simulink model "SIRVHDB_MPC_model"  (R2025a)
settings: Solver=VariableStepAuto  StartTime=0.0  StopTime=1500  RelTol=1e-3
values from neighbouring files (symbols this model uses):
  beta1 = 0.45    [SIRVDB_model_parameters.m]
  beta2 = 0.45    [SIRVDB_model_parameters.m]
  epsilon = 0.6    [SIRVDB_model_parameters.m]
  eta = 0.6    [SIRVDB_model_parameters.m]
  gamma = 1/12    (= 0.0833333333333)    [SIRVDB_model_parameters.m]
  gamma_h = 1/25    (= 0.04)    [SIRVDB_model_parameters.m]
  gamma_v = 1/9    (= 0.111111111111)    [SIRVDB_model_parameters.m]
  h = 0.05    [SIRVDB_model_parameters.m]
  H_cap1 = 0.005    [SIRVDB_model_parameters.m]
  H_cap2 = 0.005    [SIRVDB_model_parameters.m]
  H_ref = 0.8 * (H_cap1 + H_cap2)    (= 0.008)    [SIRVDB_model_parameters.m]
  h_v = 0.02    [SIRVDB_model_parameters.m]
  k = 0.7    [SIRVDB_model_parameters.m]
  M11 = 0.85    [SIRVDB_model_parameters.m]
  M12 = 0.15    [SIRVDB_model_parameters.m]
  M21 = 0.10    (= 0.1)    [SIRVDB_model_parameters.m]
  M22 = 0.90    (= 0.9)    [SIRVDB_model_parameters.m]
  mu = 0.001    [SIRVDB_model_parameters.m]
  mu_h = 0.02    [SIRVDB_model_parameters.m]
  mu_v = 0.0005    [SIRVDB_model_parameters.m]
  nu1 = 0    [SIRVDB_model_parameters.m]
  nu2 = 0    [SIRVDB_model_parameters.m]
  omega_R = 1/110    (= 0.00909090909091)    [SIRVDB_model_parameters.m]
  omega_V = 1/140    (= 0.00714285714286)    [SIRVDB_model_parameters.m]
  season_amp = 0.4    [SIRVDB_model_parameters.m]
  season_period = 365    [SIRVDB_model_parameters.m]
  travel = [-0.02  0.02 ... (first row only)    [SIRVDB_model_parameters.m]
  u1 = 0    [SIRVDB_model_parameters.m]
  u2 = 0    [SIRVDB_model_parameters.m]
libraries: mpclib x1
settings Model: Creator=Hakon  LastModifiedBy=welde
settings RTWCC: GPUComputeCapability=3.5

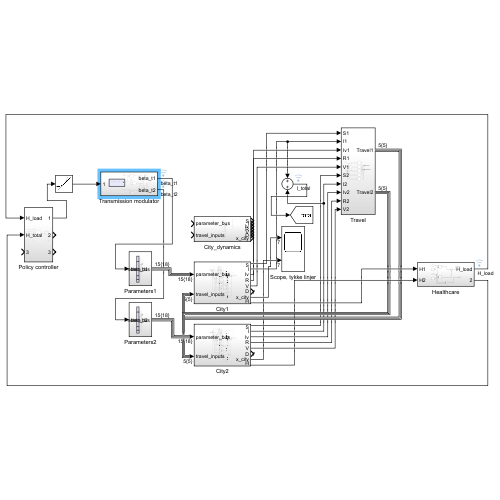
[thumbnail: Simulink's stored preview of the top-level diagram]
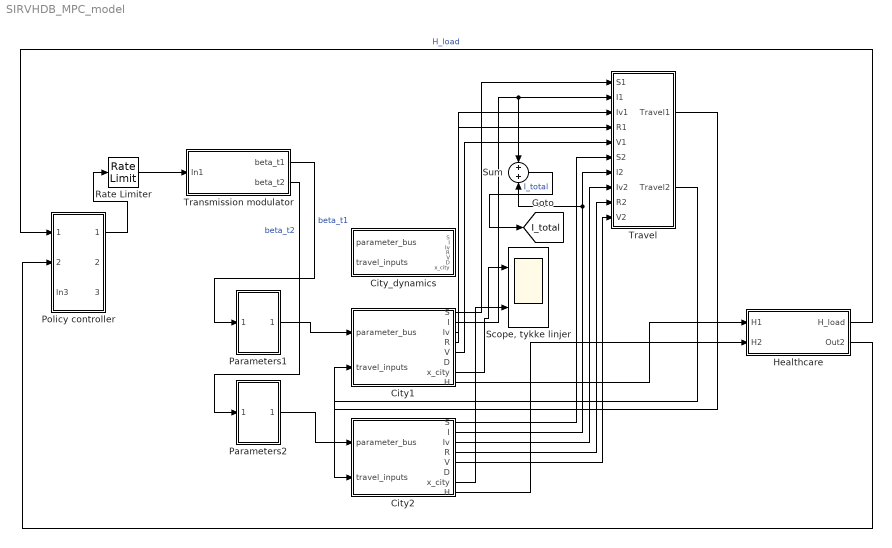
== system SIRVHDB_MPC_model ==
  City1 : Subsystem
  City2 : Subsystem
  City_dynamics : Subsystem
  Healthcare : Subsystem
  Parameters1 : Subsystem
  Parameters2 : Subsystem
  Policy controller : Subsystem
  Rate Limiter : RateLimiter  RisingSlewLimit=0.05  FallingSlewLimit=-0.05  SampleTimeMode=inherited
  "Scope, tykke linjer" : Scope  NumInputPorts=2
      settings: ActiveDisplayYMinimum=-0.125  ActiveDisplayYMaximum=1.125
  Sum : Sum
  Transmission modulator : Subsystem
  Travel : Subsystem
  tag scope: I_total=global
  wires:
  Parameters1/1(parameter_bus) -> City1/1(parameter_bus)
  City1/7(x_city) -> "Scope, tykke linjer"/1
  City2/7(x_city) -> "Scope, tykke linjer"/2
  Parameters2/1(parameter_bus) -> City2/1(parameter_bus)
  City1/1(S) -> Travel/1(S1)
  City1/2(I) -> Travel/2(I1), Sum/1
  City1/3(Iv) -> Travel/3(Iv1)
  City1/4(R) -> Travel/4(R1)
  City1/5(V) -> Travel/5(V1)
  City2/1(S) -> Travel/6(S2)
  City2/2(I) -> Travel/7(I2), Sum/2
  City2/3(Iv) -> Travel/8(Iv2)
  City2/4(R) -> Travel/9(R2)
  City2/5(V) -> Travel/10(V2)
  Travel/1(Travel1) -> City1/2(travel_inputs)
  Travel/2(Travel2) -> City2/2(travel_inputs)
  City1/8(H) -> Healthcare/1(H1)
  City2/8(H) -> Healthcare/2(H2)
  Healthcare/1(H_load) -> Policy controller/1(H_load)  "H_load"
  Transmission modulator/1(beta_t1) -> Parameters1/1(beta_t1)  "beta_t1"
  Transmission modulator/2(beta_t2) -> Parameters2/1(beta_t2)  "beta_t2"
  Healthcare/2(Out2) -> Policy controller/2(H_total)
  Policy controller/1(Out1) -> Rate Limiter/1
  Rate Limiter/1 -> Transmission modulator/1(In1)
  Sum/1 -> [I_total]  "I_total"

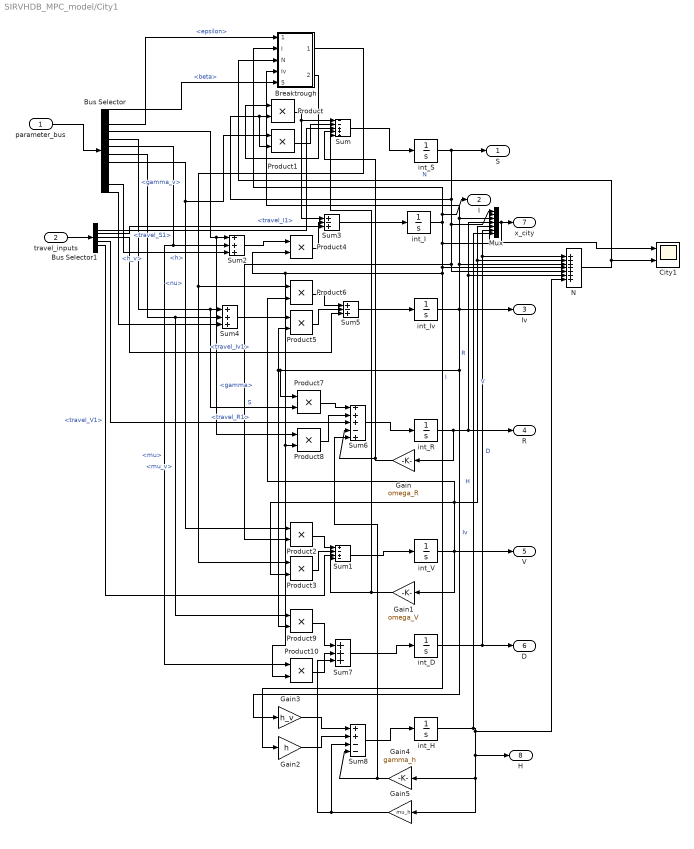
== system SIRVHDB_MPC_model/City1 ==
  parameter_bus : Inport
  travel_inputs : Inport  Port=2
  Breaktrough : Subsystem
  Bus Selector : BusSelector  OutputSignals=beta,eta,epsilon,gamma,gamma_v,mu,mu_v,nu,omega_V,omega_R,h,h_v
  Bus Selector1 : BusSelector  OutputSignals=travel_S1,travel_I1,travel_Iv1,travel_R1,travel_V1
  City1 : Scope  NumInputPorts=2
      settings: ActiveDisplayYMinimum=-0.12499999999999997  ActiveDisplayYMaximum=1.125
  Gain : Gain  Gain=omega_R
  Gain1 : Gain  Gain=omega_V
  Gain2 : Gain  Gain=h
  Gain3 : Gain  Gain=h_v
  Gain4 : Gain  Gain=gamma_h
  Gain5 : Gain  Gain=mu_h
  Mux : Mux  Inputs=7
  N : Sum  Inputs=+++++++
  Product{,1..10} (11 alike) : Product
  Sum : Sum  Inputs=--+++
  Sum1 : Sum  Inputs=+-+-
  Sum2 : Sum  Inputs=+++
  Sum3 : Sum  Inputs=+-+
  Sum4 : Sum  Inputs=+++
  Sum5 : Sum  Inputs=+-+
  Sum6 : Sum  Inputs=+++-+
  Sum7 : Sum  Inputs=+++
  Sum8 : Sum  Inputs=++--
  int_D : Integrator
  int_H : Integrator
  int_I : Integrator  InitialCondition=0.01
  int_Iv : Integrator
  int_R : Integrator
  int_S : Integrator  InitialCondition=0.99
  int_V : Integrator
  S : Outport
  I : Outport  Port=2
  Iv : Outport  Port=3
  R : Outport  Port=4
  V : Outport  Port=5
  D : Outport  Port=6
  x_city : Outport  Port=7
  H : Outport  Port=8
  wires:
  int_S/1 -> S/1, Product2/2, N/5, Mux/1, Product1/2, Product/2  "S"
  int_I/1 -> Gain2/1, Product8/2, Product10/2, Product4/2, N/4, Mux/2, I/1, Breaktrough/2(I)  "I"
  int_Iv/1 -> Gain3/1, Product9/2, Product5/2, Product7/1, Iv/1, Breaktrough/4(Iv), Mux/3, N/3  "Iv"
  int_R/1 -> Gain/1, R/1, N/6, Mux/4  "R"
  int_V/1 -> Gain1/1, V/1, Product6/2, Product3/2, Mux/5, N/2  "V"
  int_D/1 -> D/1, Mux/6, N/1  "D"
  Mux/1 -> City1/1, x_city/1
  parameter_bus/1 -> Bus Selector/1
  Bus Selector/3 -> Breaktrough/1(<epsilon>)  "<epsilon>"
  N/1 -> City1/2, Breaktrough/3(N)  "N"
  Breaktrough/2(lambda) -> Product/1
  Bus Selector/8 -> Product2/1, Product1/1  "<nu>"
  Product/1 -> Sum3/1, Sum/1
  Product1/1 -> Sum/2
  Sum/1 -> int_S/1
  Breaktrough/1(lambda_v) -> Product6/1, Product3/1
  Product2/1 -> Sum1/1
  Product3/1 -> Sum1/2
  Sum1/1 -> int_V/1
  Bus Selector/7 -> Product9/1, Sum4/2  "<mu_v>"
  Bus Selector/4 -> Product8/1, Sum2/1  "<gamma>"
  Sum2/1 -> Product4/1
  Product4/1 -> Sum3/2
  Sum3/1 -> int_I/1
  Bus Selector/5 -> Product7/2, Sum4/1  "<gamma_v>"
  Bus Selector/6 -> Product10/1, Sum2/2  "<mu>"
  Product5/1 -> Sum5/2
  Sum4/1 -> Product5/1
  Product6/1 -> Sum5/1
  Sum5/1 -> int_Iv/1
  Sum6/1 -> int_R/1
  Product7/1 -> Sum6/1
  Product8/1 -> Sum6/2
  Product9/1 -> Sum7/1
  Product10/1 -> Sum7/2
  Sum7/1 -> int_D/1
  travel_inputs/1 -> Bus Selector1/1
  Bus Selector1/1 -> Sum/3  "<travel_S1>"
  Bus Selector1/2 -> Sum3/3  "<travel_I1>"
  Bus Selector1/3 -> Sum5/3  "<travel_Iv1>"
  Bus Selector1/4 -> Sum6/3  "<travel_R1>"
  Bus Selector1/5 -> Sum1/3  "<travel_V1>"
  Gain/1 -> Sum/4, Sum6/4
  Gain1/1 -> Sum1/4, Sum/5
  int_H/1 -> Mux/7, N/7, H/1, Gain5/1, Gain4/1  "H"
  Sum8/1 -> int_H/1
  Gain2/1 -> Sum8/2
  Gain3/1 -> Sum8/1
  Gain4/1 -> Sum6/5, Sum8/4
  Gain5/1 -> Sum7/3, Sum8/3
  Bus Selector/11 -> Sum2/3  "<h>"
  Bus Selector/12 -> Sum4/3  "<h_v>"
  Bus Selector/1 -> Breaktrough/5(<beta>)  "<beta>"

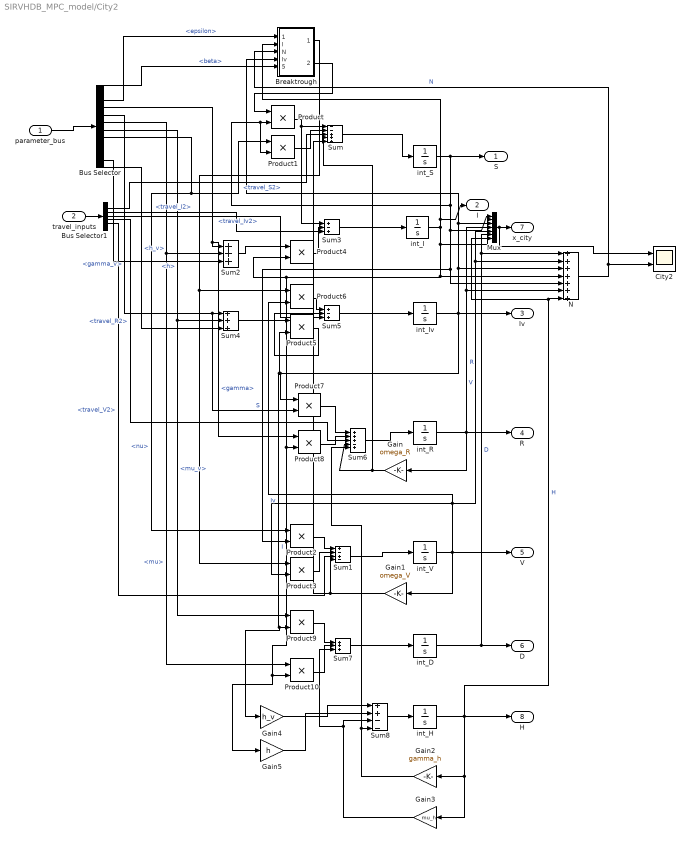
== system SIRVHDB_MPC_model/City2 ==
  parameter_bus : Inport
  travel_inputs : Inport  Port=2
  Breaktrough : Subsystem
  Bus Selector : BusSelector  OutputSignals=beta,eta,epsilon,gamma,gamma_v,mu,mu_v,nu,omega_V,omega_R,h,h_v
  Bus Selector1 : BusSelector  OutputSignals=travel_S2,travel_I2,travel_Iv2,travel_R2,travel_V2
  City2 : Scope  NumInputPorts=2
      settings: ActiveDisplayYMinimum=-0.125  ActiveDisplayYMaximum=1.125
  Gain : Gain  Gain=omega_R
  Gain1 : Gain  Gain=omega_V
  Gain2 : Gain  Gain=gamma_h
  Gain3 : Gain  Gain=mu_h
  Gain4 : Gain  Gain=h_v
  Gain5 : Gain  Gain=h
  Mux : Mux  Inputs=7
  N : Sum  Inputs=+++++++
  Product{,1..10} (11 alike) : Product
  Sum : Sum  Inputs=--+++
  Sum1 : Sum  Inputs=+-+-
  Sum2 : Sum  Inputs=+++
  Sum3 : Sum  Inputs=+-+
  Sum4 : Sum  Inputs=+++
  Sum5 : Sum  Inputs=+-+
  Sum6 : Sum  Inputs=+++-+
  Sum7 : Sum  Inputs=+++
  Sum8 : Sum  Inputs=++--
  int_D : Integrator
  int_H : Integrator
  int_I : Integrator  InitialCondition=0.01
  int_Iv : Integrator
  int_R : Integrator
  int_S : Integrator  InitialCondition=0.99
  int_V : Integrator
  S : Outport
  I : Outport  Port=2
  Iv : Outport  Port=3
  R : Outport  Port=4
  V : Outport  Port=5
  D : Outport  Port=6
  x_city : Outport  Port=7
  H : Outport  Port=8
  wires:
  int_S/1 -> S/1, Product2/2, N/5, Mux/1, Product1/2, Product/2  "S"
  int_I/1 -> Product8/2, Gain5/1, Product10/2, Product4/2, N/4, Mux/2, I/1, Breaktrough/2(I)  "I"
  int_Iv/1 -> Iv/1, Gain4/1, Product9/2, Product5/2, Product7/1, Breaktrough/4(Iv), Mux/3, N/3  "Iv"
  int_R/1 -> Gain/1, R/1, Mux/4, N/6  "R"
  int_V/1 -> Gain1/1, V/1, Product6/2, Product3/2, Mux/5, N/2  "V"
  int_D/1 -> D/1, Mux/6, N/1  "D"
  Mux/1 -> City2/1, x_city/1
  parameter_bus/1 -> Bus Selector/1
  Bus Selector/3 -> Breaktrough/1(<epsilon>)  "<epsilon>"
  N/1 -> City2/2, Breaktrough/3(N)  "N"
  Breaktrough/2(lambda) -> Product/1
  Bus Selector/8 -> Product2/1, Product1/1  "<nu>"
  Product/1 -> Sum3/1, Sum/1
  Product1/1 -> Sum/2
  Breaktrough/1(lambda_v) -> Product6/1, Product3/1
  Product2/1 -> Sum1/1
  Product3/1 -> Sum1/2
  Sum1/1 -> int_V/1
  Bus Selector/7 -> Product9/1, Sum4/2  "<mu_v>"
  Bus Selector/4 -> Product8/1, Sum2/1  "<gamma>"
  Sum2/1 -> Product4/1
  Product4/1 -> Sum3/2
  Sum3/1 -> int_I/1
  Bus Selector/5 -> Product7/2, Sum4/1  "<gamma_v>"
  Bus Selector/6 -> Product10/1, Sum2/2  "<mu>"
  Product5/1 -> Sum5/2
  Sum4/1 -> Product5/1
  Product6/1 -> Sum5/1
  Sum5/1 -> int_Iv/1
  Sum6/1 -> int_R/1
  Product7/1 -> Sum6/1
  Product8/1 -> Sum6/2
  Product9/1 -> Sum7/1
  Product10/1 -> Sum7/2
  Sum7/1 -> int_D/1
  travel_inputs/1 -> Bus Selector1/1
  Bus Selector1/1 -> Sum/3  "<travel_S2>"
  Bus Selector1/2 -> Sum3/3  "<travel_I2>"
  Bus Selector1/3 -> Sum5/3  "<travel_Iv2>"
  Bus Selector1/4 -> Sum6/3  "<travel_R2>"
  Bus Selector1/5 -> Sum1/3  "<travel_V2>"
  Gain/1 -> Sum6/4, Sum/4
  Gain1/1 -> Sum/5, Sum1/4
  Bus Selector/11 -> Sum2/3  "<h>"
  Bus Selector/12 -> Sum4/3  "<h_v>"
  int_H/1 -> Mux/7, N/7, H/1, Gain3/1, Gain2/1  "H"
  Sum8/1 -> int_H/1
  Gain2/1 -> Sum6/5, Sum8/4
  Gain3/1 -> Sum7/3, Sum8/3
  Gain4/1 -> Sum8/1
  Gain5/1 -> Sum8/2
  Bus Selector/1 -> Breaktrough/5(beta_t2)  "<beta>"
  Sum/1 -> int_S/1

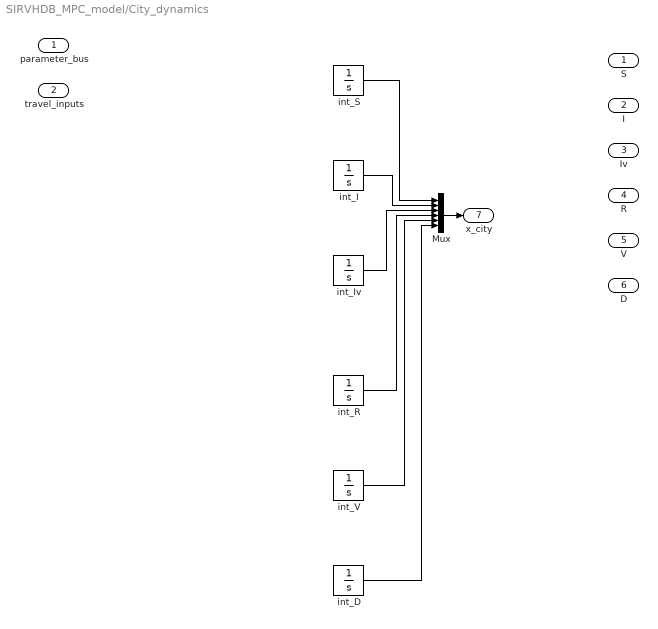
== system SIRVHDB_MPC_model/City_dynamics ==
  parameter_bus : Inport
  travel_inputs : Inport  Port=2
  Mux : Mux  Inputs=6
  int_D : Integrator
  int_I : Integrator  InitialCondition=0.01
  int_Iv : Integrator
  int_R : Integrator
  int_S : Integrator  InitialCondition=0.99
  int_V : Integrator
  S : Outport
  I : Outport  Port=2
  Iv : Outport  Port=3
  R : Outport  Port=4
  V : Outport  Port=5
  D : Outport  Port=6
  x_city : Outport  Port=7
  wires:
  int_S/1 -> Mux/1
  int_I/1 -> Mux/2
  int_Iv/1 -> Mux/3
  int_R/1 -> Mux/4
  int_V/1 -> Mux/5
  int_D/1 -> Mux/6
  Mux/1 -> x_city/1

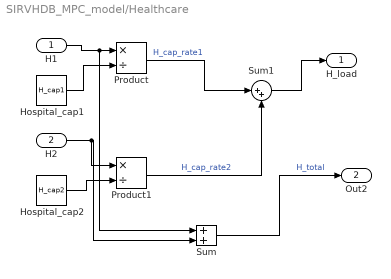
== system SIRVHDB_MPC_model/Healthcare ==
  H1 : Inport
  H2 : Inport  Port=2
  Hospital_cap1 : Constant  Value=H_cap1
  Hospital_cap2 : Constant  Value=H_cap2
  Product : Product  Inputs=*/
  Product1 : Product  Inputs=*/
  Sum : Sum
  Sum1 : Sum  Inputs=|++
  H_load : Outport
  Out2 : Outport  Port=2
  wires:
  H2/1 -> Sum/2, Product1/1
  Hospital_cap2/1 -> Product1/2
  H1/1 -> Sum/1, Product/1
  Hospital_cap1/1 -> Product/2
  Product/1 -> Sum1/1  "H_cap_rate1"
  Product1/1 -> Sum1/2  "H_cap_rate2"
  Sum1/1 -> H_load/1
  Sum/1 -> Out2/1  "H_total"

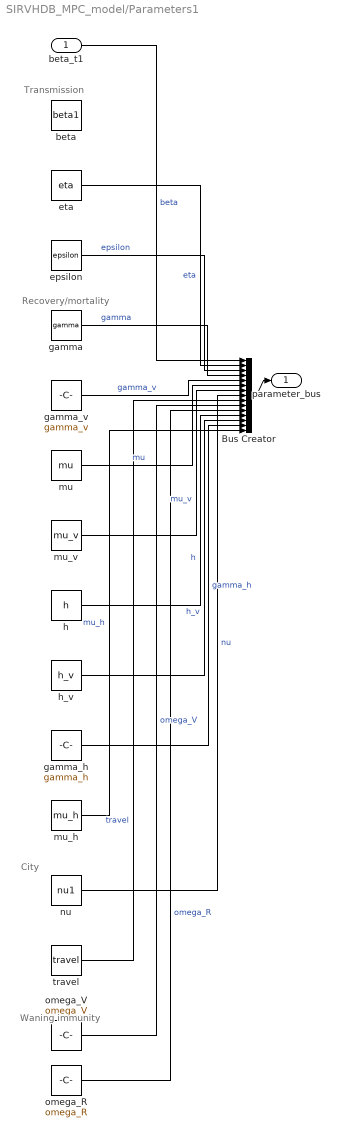
== system SIRVHDB_MPC_model/Parameters1 ==
  note: Waning immunity
  note: Transmission
  note: City
  note: Recovery/mortality
  beta_t1 : Inport
  Bus Creator : BusCreator  Inputs=15
  beta : Constant  Value=beta1  SampleTime=-1
  epsilon : Constant  Value=epsilon  SampleTime=-1
  eta : Constant  Value=eta  SampleTime=-1
  gamma : Constant  Value=gamma  SampleTime=-1
  gamma_h : Constant  Value=gamma_h  SampleTime=-1
  gamma_v : Constant  Value=gamma_v  SampleTime=-1
  h : Constant  Value=h  SampleTime=-1
  h_v : Constant  Value=h_v  SampleTime=-1
  mu : Constant  Value=mu  SampleTime=-1
  mu_h : Constant  Value=mu_h  SampleTime=-1
  mu_v : Constant  Value=mu_v  SampleTime=-1
  nu : Constant  Value=nu1  SampleTime=-1
  omega_R : Constant  Value=omega_R  SampleTime=-1
  omega_V : Constant  Value=omega_V  SampleTime=-1
  travel : Constant  Value=travel  SampleTime=-1
  parameter_bus : Outport
  wires:
  travel/1 -> Bus Creator/9  "travel"
  mu_v/1 -> Bus Creator/7  "mu_v"
  Bus Creator/1 -> parameter_bus/1
  epsilon/1 -> Bus Creator/3  "epsilon"
  eta/1 -> Bus Creator/2  "eta"
  gamma/1 -> Bus Creator/4  "gamma"
  nu/1 -> Bus Creator/8  "nu"
  gamma_v/1 -> Bus Creator/5  "gamma_v"
  mu/1 -> Bus Creator/6  "mu"
  omega_V/1 -> Bus Creator/10  "omega_V"
  omega_R/1 -> Bus Creator/11  "omega_R"
  beta_t1/1 -> Bus Creator/1  "beta"
  h/1 -> Bus Creator/12  "h"
  h_v/1 -> Bus Creator/13  "h_v"
  gamma_h/1 -> Bus Creator/14  "gamma_h"
  mu_h/1 -> Bus Creator/15  "mu_h"

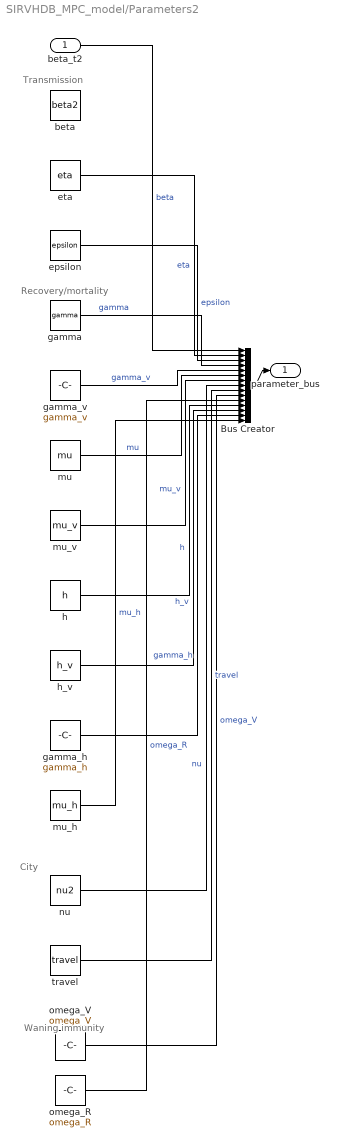
== system SIRVHDB_MPC_model/Parameters2 ==
  note: Transmission
  note: City
  note: Recovery/mortality
  note: Waning immunity
  beta_t2 : Inport
  Bus Creator : BusCreator  Inputs=15
  beta : Constant  Value=beta2  SampleTime=-1
  epsilon : Constant  Value=epsilon  SampleTime=-1
  eta : Constant  Value=eta  SampleTime=-1
  gamma : Constant  Value=gamma  SampleTime=-1
  gamma_h : Constant  Value=gamma_h  SampleTime=-1
  gamma_v : Constant  Value=gamma_v  SampleTime=-1
  h : Constant  Value=h  SampleTime=-1
  h_v : Constant  Value=h_v  SampleTime=-1
  mu : Constant  Value=mu  SampleTime=-1
  mu_h : Constant  Value=mu_h  SampleTime=-1
  mu_v : Constant  Value=mu_v  SampleTime=-1
  nu : Constant  Value=nu2  SampleTime=-1
  omega_R : Constant  Value=omega_R  SampleTime=-1
  omega_V : Constant  Value=omega_V  SampleTime=-1
  travel : Constant  Value=travel  SampleTime=-1
  parameter_bus : Outport
  wires:
  travel/1 -> Bus Creator/9  "travel"
  mu_v/1 -> Bus Creator/7  "mu_v"
  Bus Creator/1 -> parameter_bus/1
  epsilon/1 -> Bus Creator/3  "epsilon"
  eta/1 -> Bus Creator/2  "eta"
  gamma/1 -> Bus Creator/4  "gamma"
  nu/1 -> Bus Creator/8  "nu"
  gamma_v/1 -> Bus Creator/5  "gamma_v"
  mu/1 -> Bus Creator/6  "mu"
  omega_V/1 -> Bus Creator/10  "omega_V"
  omega_R/1 -> Bus Creator/11  "omega_R"
  beta_t2/1 -> Bus Creator/1  "beta"
  h/1 -> Bus Creator/12  "h"
  h_v/1 -> Bus Creator/13  "h_v"
  gamma_h/1 -> Bus Creator/14  "gamma_h"
  mu_h/1 -> Bus Creator/15  "mu_h"

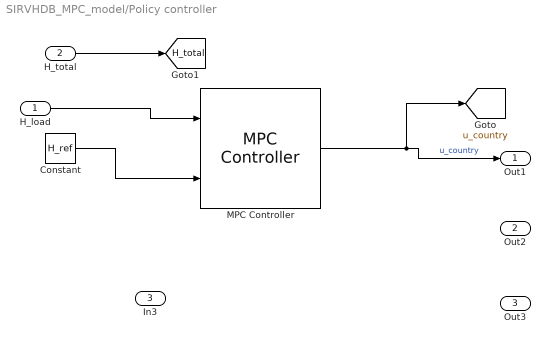
== system SIRVHDB_MPC_model/Policy controller ==
  H_load : Inport
  H_total : Inport  Port=2
  In3 : Inport  Port=3
  Constant : Constant  Value=H_ref  SampleTime=-1
  MPC Controller : mpclib/MPC Controller  SCDEnableBlockLinearizationSpecification=on  mpcobj=mpcobj  x0=xmpc  is_multiple=0  enable_value=0  return_u0=off  updateMPCinCallerWorkspace=on  md_inport=off  mv_inport=off  uref_inport=off  return_cost=off  return_mvseq=off  return_qpstatus=off  return_xseq=off  return_state=off  return_ovseq=off  state_inport=off  umin_inport=off  umax_inport=off  ymin_inport=off  ymax_inport=off  cc_inport=off  ywt_inport=off  uwt_inport=off  duwt_inport=off  rhoeps_inport=off  pm_inport=off  MaximumP=10  HorizonChoice=FixedHorizon  n_ts=1  n_p=40  n_mv=1  n_md=0  n_ud=0  n_mo=1  n_uo=0  BlockDataType=double  SampleTimeInherited=off  switch_inport=off
  Out1 : Outport
  Out2 : Outport  Port=2
  Out3 : Outport  Port=3
  tag scope: H_total=global, u_country=global
  wires:
  ? -> Out2/1
  ? -> Out3/1
  H_total/1 -> [H_total]
  H_load/1 -> MPC Controller/1
  MPC Controller/1 -> [u_country], Out1/1  "u_country"
  Constant/1 -> MPC Controller/2

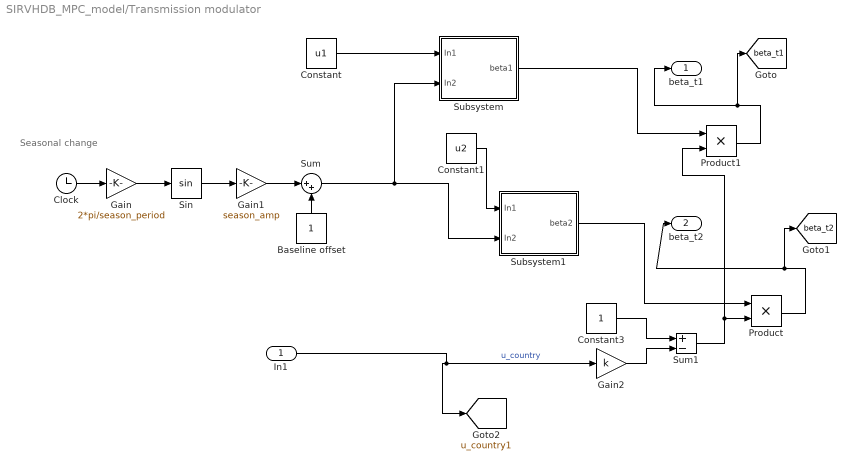
== system SIRVHDB_MPC_model/Transmission modulator ==
  note: Seasonal change
  In1 : Inport
  Baseline offset : Constant  SampleTime=-1
  Clock : Clock
  Constant : Constant  Value=u1
  Constant1 : Constant  Value=u2
  Constant3 : Constant
  Gain : Gain  Gain=2*pi/season_period
  Gain1 : Gain  Gain=season_amp
  Gain2 : Gain  Gain=k
  Product : Product
  Product1 : Product
  Sin : Trigonometry
  Subsystem : Subsystem
  Subsystem1 : Subsystem
  Sum : Sum  Inputs=|++
  Sum1 : Sum  Inputs=+-
  beta_t1 : Outport
  beta_t2 : Outport  Port=2
  tag scope: beta_t1=global, beta_t2=global, u_country1=global
  wires:
  Gain1/1 -> Sum/1
  Baseline offset/1 -> Sum/2
  Gain/1 -> Sin/1
  Sin/1 -> Gain1/1
  Clock/1 -> Gain/1
  Constant/1 -> Subsystem/1(In1)
  Sum/1 -> Subsystem1/2(In2), Subsystem/2(In2)
  Subsystem/1(beta1) -> Product1/1
  Constant1/1 -> Subsystem1/1(In1)
  Subsystem1/1(beta2) -> Product/1
  In1/1 -> Gain2/1, [u_country1]  "u_country"
  Gain2/1 -> Sum1/2
  Constant3/1 -> Sum1/1
  Sum1/1 -> Product1/2, Product/2
  Product/1 -> [beta_t2], beta_t2/1
  Product1/1 -> [beta_t1], beta_t1/1

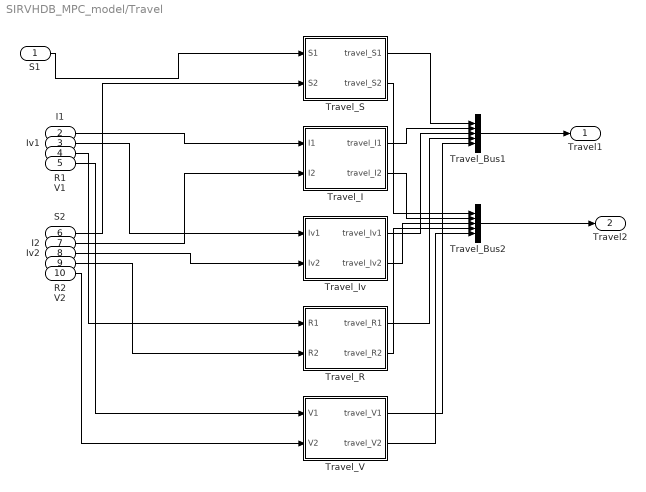
== system SIRVHDB_MPC_model/Travel ==
  S1 : Inport
  I1 : Inport  Port=2
  Iv1 : Inport  Port=3
  R1 : Inport  Port=4
  V1 : Inport  Port=5
  S2 : Inport  Port=6
  I2 : Inport  Port=7
  Iv2 : Inport  Port=8
  R2 : Inport  Port=9
  V2 : Inport  Port=10
  Travel_Bus1 : BusCreator  Inputs=5
  Travel_Bus2 : BusCreator  Inputs=5
  Travel_I : Subsystem
  Travel_Iv : Subsystem
  Travel_R : Subsystem
  Travel_S : Subsystem
  Travel_V : Subsystem
  Travel1 : Outport
  Travel2 : Outport  Port=2
  wires:
  Travel_Bus2/1 -> Travel2/1
  V1/1 -> Travel_V/1(V1)
  S2/1 -> Travel_S/2(S2)
  V2/1 -> Travel_V/2(V2)
  Iv1/1 -> Travel_Iv/1(Iv1)
  Travel_V/2(travel_V2) -> Travel_Bus2/5
  Travel_Iv/2(travel_Iv2) -> Travel_Bus2/3
  Travel_I/2(travel_I2) -> Travel_Bus2/2
  Travel_R/2(travel_R2) -> Travel_Bus2/4
  I1/1 -> Travel_I/1(I1)
  Travel_I/1(travel_I1) -> Travel_Bus1/2
  I2/1 -> Travel_I/2(I2)
  Iv2/1 -> Travel_Iv/2(Iv2)
  Travel_Bus1/1 -> Travel1/1
  Travel_S/1(travel_S1) -> Travel_Bus1/1
  R1/1 -> Travel_R/1(R1)
  Travel_Iv/1(travel_Iv1) -> Travel_Bus1/3
  R2/1 -> Travel_R/2(R2)
  Travel_S/2(travel_S2) -> Travel_Bus2/1
  Travel_R/1(travel_R1) -> Travel_Bus1/4
  Travel_V/1(travel_V1) -> Travel_Bus1/5
  S1/1 -> Travel_S/1(S1)

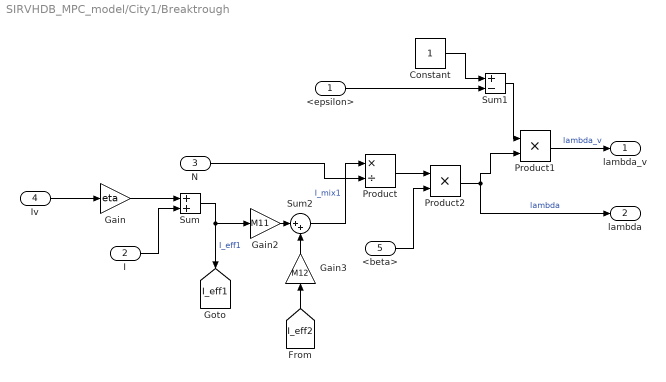
== system SIRVHDB_MPC_model/City1/Breaktrough ==
  <epsilon> : Inport
  I : Inport  Port=2
  N : Inport  Port=3
  Iv : Inport  Port=4
  <beta> : Inport  Port=5
  Constant : Constant
  Gain : Gain  Gain=eta
  Gain2 : Gain  Gain=M11
  Gain3 : Gain  Gain=M12
  Product : Product  Inputs=*/
  Product1 : Product
  Product2 : Product
  Sum : Sum
  Sum1 : Sum  Inputs=+-
  Sum2 : Sum  Inputs=|++
  lambda_v : Outport
  lambda : Outport  Port=2
  tag scope: I_eff1=global
  wires:
  Product1/1 -> lambda_v/1  "lambda_v"
  <epsilon>/1 -> Sum1/2
  Gain/1 -> Sum/1
  I/1 -> Sum/2
  Product2/1 -> Product1/2, lambda/1  "lambda"
  Constant/1 -> Sum1/1
  Product/1 -> Product2/1
  N/1 -> Product/2
  Sum/1 -> [I_eff1], Gain2/1  "I_eff1"
  Iv/1 -> Gain/1
  Sum1/1 -> Product1/1
  [I_eff2] -> Gain3/1
  Gain2/1 -> Sum2/1
  Gain3/1 -> Sum2/2
  Sum2/1 -> Product/1  "I_mix1"
  <beta>/1 -> Product2/2

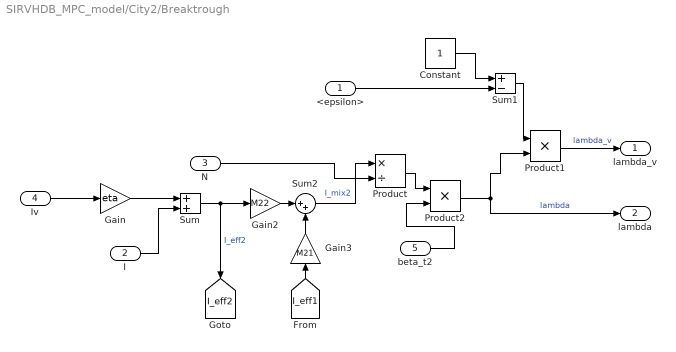
== system SIRVHDB_MPC_model/City2/Breaktrough ==
  <epsilon> : Inport
  I : Inport  Port=2
  N : Inport  Port=3
  Iv : Inport  Port=4
  beta_t2 : Inport  Port=5
  Constant : Constant
  Gain : Gain  Gain=eta
  Gain2 : Gain  Gain=M22
  Gain3 : Gain  Gain=M21
  Product : Product  Inputs=*/
  Product1 : Product
  Product2 : Product
  Sum : Sum
  Sum1 : Sum  Inputs=+-
  Sum2 : Sum  Inputs=|++
  lambda_v : Outport
  lambda : Outport  Port=2
  tag scope: I_eff2=global
  wires:
  Product1/1 -> lambda_v/1  "lambda_v"
  <epsilon>/1 -> Sum1/2
  Gain/1 -> Sum/1
  I/1 -> Sum/2
  Product2/1 -> lambda/1, Product1/2  "lambda"
  Constant/1 -> Sum1/1
  Product/1 -> Product2/1
  N/1 -> Product/2
  Sum/1 -> Gain2/1, [I_eff2]  "I_eff2"
  Iv/1 -> Gain/1
  Sum1/1 -> Product1/1
  [I_eff1] -> Gain3/1
  Gain2/1 -> Sum2/1
  Gain3/1 -> Sum2/2
  Sum2/1 -> Product/1  "I_mix2"
  beta_t2/1 -> Product2/2

== system SIRVHDB_MPC_model/Transmission modulator/Subsystem ==
  In1 : Inport
  In2 : Inport  Port=2
  Constant1 : Constant
  Gain2 : Gain  Gain=beta1
  Gain3 : Gain  Gain=k
  Product : Product
  Sum1 : Sum  Inputs=+-
  beta1 : Outport
  wires:
  In2/1 -> Gain2/1
  Sum1/1 -> Product/1
  Constant1/1 -> Sum1/1
  Gain3/1 -> Sum1/2
  In1/1 -> Gain3/1
  Gain2/1 -> Product/2, beta1/1  "beta_t1"
  Product/1 -> ?  "beta_controlled1"

== system SIRVHDB_MPC_model/Transmission modulator/Subsystem1 ==
  In1 : Inport
  In2 : Inport  Port=2
  Constant1 : Constant
  Gain2 : Gain  Gain=beta2
  Gain3 : Gain  Gain=k
  Product : Product
  Sum1 : Sum  Inputs=+-
  beta2 : Outport
  wires:
  In2/1 -> Gain2/1
  Sum1/1 -> Product/1
  Constant1/1 -> Sum1/1
  Gain3/1 -> Sum1/2
  In1/1 -> Gain3/1
  Gain2/1 -> Product/2, beta2/1  "beta_t1"
  Product/1 -> ?  "beta_controlled2"

== system SIRVHDB_MPC_model/Travel/Travel_I ==
  I1 : Inport
  I2 : Inport  Port=2
  Constant : Constant  Value=travel  SampleTime=-1
  Matrix Multiply : Product  Inputs=**  Multiplication=Matrix(*)
  Selector : Selector  InputPortWidth=2  IndexOptions=Index vector (dialog)  Indices=[1]  OutputSizes=1
  Selector1 : Selector  InputPortWidth=2  IndexOptions=Index vector (dialog)  Indices=[2]  OutputSizes=1
  Vector Concatenate : Concatenate
  travel_I1 : Outport
  travel_I2 : Outport  Port=2
  wires:
  Selector1/1 -> travel_I2/1  "travel_I2"
  Matrix Multiply/1 -> Selector1/1, Selector/1
  I1/1 -> Vector Concatenate/1
  Constant/1 -> Matrix Multiply/1
  Selector/1 -> travel_I1/1  "travel_I1"
  I2/1 -> Vector Concatenate/2
  Vector Concatenate/1 -> Matrix Multiply/2

== system SIRVHDB_MPC_model/Travel/Travel_Iv ==
  Iv1 : Inport
  Iv2 : Inport  Port=2
  Constant : Constant  Value=travel  SampleTime=-1
  Matrix Multiply : Product  Inputs=**  Multiplication=Matrix(*)
  Selector : Selector  InputPortWidth=2  IndexOptions=Index vector (dialog)  Indices=[1]  OutputSizes=1
  Selector1 : Selector  InputPortWidth=2  IndexOptions=Index vector (dialog)  Indices=[2]  OutputSizes=1
  Vector Concatenate : Concatenate
  travel_Iv1 : Outport
  travel_Iv2 : Outport  Port=2
  wires:
  Selector1/1 -> travel_Iv2/1  "travel_Iv2"
  Matrix Multiply/1 -> Selector1/1, Selector/1
  Iv1/1 -> Vector Concatenate/1
  Constant/1 -> Matrix Multiply/1
  Selector/1 -> travel_Iv1/1  "travel_Iv1"
  Iv2/1 -> Vector Concatenate/2
  Vector Concatenate/1 -> Matrix Multiply/2

== system SIRVHDB_MPC_model/Travel/Travel_R ==
  R1 : Inport
  R2 : Inport  Port=2
  Constant : Constant  Value=travel  SampleTime=-1
  Matrix Multiply : Product  Inputs=**  Multiplication=Matrix(*)
  Selector : Selector  InputPortWidth=2  IndexOptions=Index vector (dialog)  Indices=[1]  OutputSizes=1
  Selector1 : Selector  InputPortWidth=2  IndexOptions=Index vector (dialog)  Indices=[2]  OutputSizes=1
  Vector Concatenate : Concatenate
  travel_R1 : Outport
  travel_R2 : Outport  Port=2
  wires:
  Selector1/1 -> travel_R2/1  "travel_R2"
  Matrix Multiply/1 -> Selector1/1, Selector/1
  R1/1 -> Vector Concatenate/1
  Constant/1 -> Matrix Multiply/1
  Selector/1 -> travel_R1/1  "travel_R1"
  R2/1 -> Vector Concatenate/2
  Vector Concatenate/1 -> Matrix Multiply/2

== system SIRVHDB_MPC_model/Travel/Travel_S ==
  S1 : Inport
  S2 : Inport  Port=2
  Constant : Constant  Value=travel  SampleTime=-1
  Matrix Multiply : Product  Inputs=**  Multiplication=Matrix(*)
  Selector : Selector  InputPortWidth=2  IndexOptions=Index vector (dialog)  Indices=[1]  OutputSizes=1
  Selector1 : Selector  InputPortWidth=2  IndexOptions=Index vector (dialog)  Indices=[2]  OutputSizes=1
  Vector Concatenate : Concatenate
  travel_S1 : Outport
  travel_S2 : Outport  Port=2
  wires:
  Selector1/1 -> travel_S2/1  "travel_S2"
  Matrix Multiply/1 -> Selector1/1, Selector/1
  S1/1 -> Vector Concatenate/1
  Constant/1 -> Matrix Multiply/1
  Selector/1 -> travel_S1/1  "travel_S1"
  S2/1 -> Vector Concatenate/2
  Vector Concatenate/1 -> Matrix Multiply/2

== system SIRVHDB_MPC_model/Travel/Travel_V ==
  V1 : Inport
  V2 : Inport  Port=2
  Constant : Constant  Value=travel  SampleTime=-1
  Matrix Multiply : Product  Inputs=**  Multiplication=Matrix(*)
  Selector : Selector  InputPortWidth=2  IndexOptions=Index vector (dialog)  Indices=[1]  OutputSizes=1
  Selector1 : Selector  InputPortWidth=2  IndexOptions=Index vector (dialog)  Indices=[2]  OutputSizes=1
  Vector Concatenate : Concatenate
  travel_V1 : Outport
  travel_V2 : Outport  Port=2
  wires:
  Selector1/1 -> travel_V2/1  "travel_V2"
  Matrix Multiply/1 -> Selector1/1, Selector/1
  V1/1 -> Vector Concatenate/1
  Constant/1 -> Matrix Multiply/1
  Selector/1 -> travel_V1/1  "travel_V1"
  V2/1 -> Vector Concatenate/2
  Vector Concatenate/1 -> Matrix Multiply/2
